simulink library "DC_GRIDSIM_LIB"  (R2022b)
settings: Solver=VariableStepAuto  StartTime=0.0  StopTime=10.0  RelTol=1e-3
undefined symbols (not defined in the file): Allday_timevector, DiscIntNeverNeededParam, High, Household1_Autumnallday, Household1_Springallday, Household1_Summerallday, Household1_Winterallday, Household9_Autumnallday, Household9_Springallday, Household9_Summerallday, Household9_Winterallday, Low, MV, Shift
libraries: fl_lib x66, nesl_utility x33, simulink x8, ee_lib x4
(part 2 of 2)

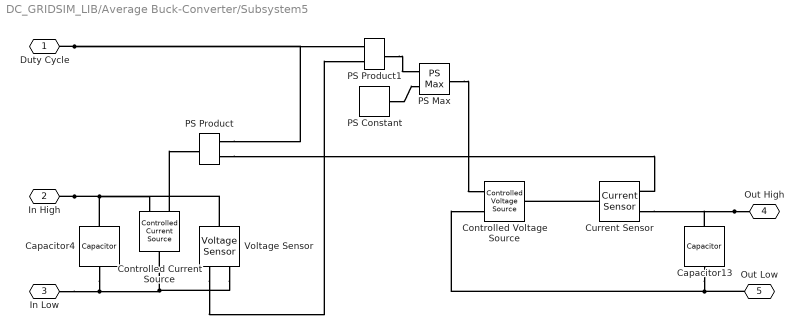
== system DC_GRIDSIM_LIB/Average Buck-Converter/Subsystem5 ==
  Capacitor13 : fl_lib/Electrical/Electrical Elements/Capacitor  c=C uF  r=1e-6 Ohm  g=0 1/Ohm  i_specify=off  i_priority=None  i=1 A  i_nominal_specify=off  i_nominal_unit=A  i_nominal_value=1  v_specify=off  v_priority=None  v=48 V  v_nominal_specify=off  v_nominal_unit=V  v_nominal_value=1  vc_specify=on  vc_priority=None  vc=LV V  vc_nominal_specify=off  vc_nominal_unit=V  vc_nominal_value=1
  Capacitor4 : fl_lib/Electrical/Electrical Elements/Capacitor  c=C uF  r=1e-6 Ohm  g=0 1/Ohm  i_specify=off  i_priority=None  i=1 A  i_nominal_specify=off  i_nominal_unit=A  i_nominal_value=1  v_specify=off  v_priority=High  v=LV V  v_nominal_specify=off  v_nominal_unit=V  v_nominal_value=1  vc_specify=on  vc_priority=None  vc=MV V  vc_nominal_specify=off  vc_nominal_unit=V  vc_nominal_value=1
  Controlled Current Source : fl_lib/Electrical/Electrical Sources/Controlled Current Source
  Controlled Voltage Source : fl_lib/Electrical/Electrical Sources/Controlled Voltage Source
  Current Sensor : fl_lib/Electrical/Electrical Sensors/Current Sensor
  PS Constant : fl_lib/Physical Signals/Sources/PS Constant  constant=1e-3 V
  PS Max : fl_lib/Physical Signals/Nonlinear Operators/PS Max
      settings: InternalSimscapePortConfiguration="{\"Bottom\":[],\"Left\":[{\"id\":\"I1\",\"label\":\"\",\"type\":\"input\"},{\"id\":\"I2\",\"label\":\"\",\"type\":\"input\"}],\"Right\":[{\"id\":\"O\",\"label\":\"\",\"type\":\"output\"}],\"Top\":[]}"
  PS Product : fl_lib/Physical Signals/Functions/PS Product
  PS Product1 : fl_lib/Physical Signals/Functions/PS Product
  Voltage Sensor : fl_lib/Electrical/Electrical Sensors/Voltage Sensor
  Duty Cycle : PMIOPort  Side=Left
  In High : PMIOPort  Port=2  Side=Left
  In Low : PMIOPort  Port=3  Side=Left
  Out High : PMIOPort  Port=4  Side=Right
  Out Low : PMIOPort  Port=5  Side=Right
  connections:
  In High/RConn1 -- Capacitor4/LConn1 -- Voltage Sensor/LConn1 -- Controlled Current Source/RConn2
  In Low/RConn1 -- Capacitor4/RConn1 -- Voltage Sensor/RConn2 -- Controlled Current Source/LConn1
  Duty Cycle/RConn1 -- PS Product/LConn2 -- PS Product1/LConn1
  Out Low/RConn1 -- Capacitor13/RConn1 -- Controlled Voltage Source/RConn2
  Out High/RConn1 -- Current Sensor/RConn2 -- Capacitor13/LConn1
  Current Sensor/LConn1 -- Controlled Voltage Source/LConn1
  PS Constant/RConn1 -- PS Max/LConn2
  Controlled Current Source/RConn1 -- PS Product/RConn1
  Voltage Sensor/RConn1 -- PS Product1/LConn2
  PS Product/LConn1 -- Current Sensor/RConn1
  PS Product1/RConn1 -- PS Max/LConn1
  PS Max/RConn1 -- Controlled Voltage Source/RConn1

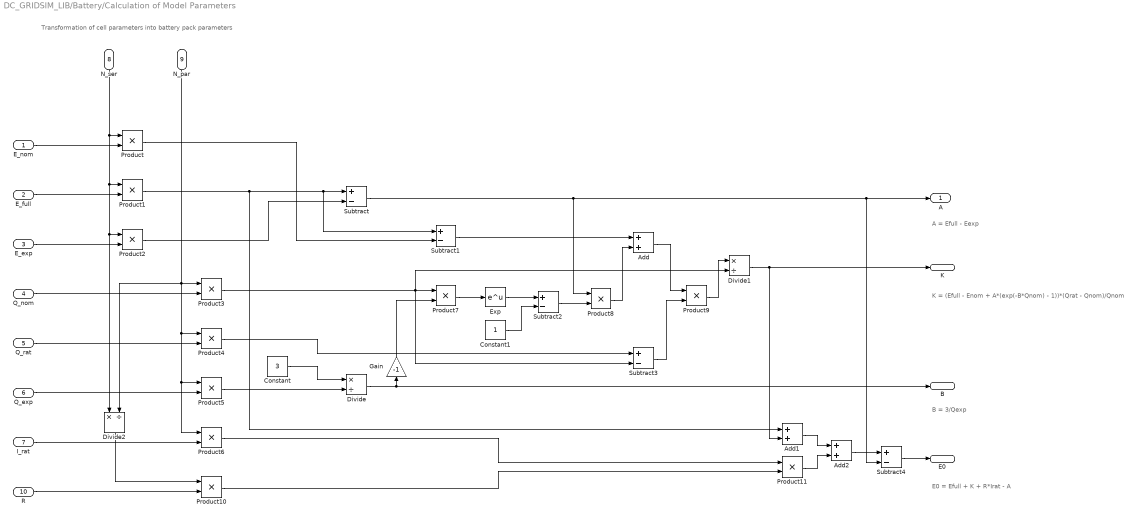
== system DC_GRIDSIM_LIB/Battery/Calculation of Model Parameters ==
  note: A = Efull - Eexp
  note: K = (Efull - Enom + A*(exp(-B*Qnom) - 1))*(Qrat - Qnom)/Qnom
  note: B = 3/Qexp
  note: E0 = Efull + K + R*Irat - A
  note: Transformation of cell parameters into battery pack parameters
  E_nom : Inport
  E_full : Inport  Port=2
  E_exp : Inport  Port=3
  Q_nom : Inport  Port=4
  Q_rat : Inport  Port=5
  Q_exp : Inport  Port=6
  I_rat : Inport  Port=7
  N_ser : Inport  Port=8
  N_par : Inport  Port=9
  R : Inport  Port=10
  Add : Sum
  Add1 : Sum
  Add2 : Sum
  Constant : Constant  Value=3
  Constant1 : Constant
  Divide : Product  Inputs=*/
  Divide1 : Product  Inputs=*/
  Divide2 : Product  Inputs=*/
  Exp : Math
  Gain : Gain  Gain=-1
  Product{,1..11} (12 alike) : Product
  Subtract{,1..4} (5 alike) : Sum  Inputs=+-
  A : Outport
  B : Outport  Port=2
  K : Outport  Port=3
  E0 : Outport  Port=4
  wires:
  Subtract4/1 -> E0/1
  Add2/1 -> Subtract4/1
  Product11/1 -> Add2/2
  Add1/1 -> Add2/1
  Product10/1 -> Product11/2
  Product6/1 -> Product11/1
  Divide2/1 -> Product10/1
  R/1 -> Product10/2
  Divide1/1 -> K/1, Add1/2
  Product9/1 -> Divide1/1
  Subtract3/1 -> Product9/2
  Add/1 -> Product9/1
  Product4/1 -> Subtract3/1
  Product8/1 -> Add/2
  Subtract2/1 -> Product8/2
  Constant1/1 -> Subtract2/2
  Exp/1 -> Subtract2/1
  Subtract1/1 -> Add/1
  Product7/1 -> Exp/1
  Product3/1 -> Product7/1, Divide1/2, Subtract3/2
  Gain/1 -> Product7/2
  Product/1 -> Subtract1/2
  Divide/1 -> Gain/1, B/1
  Product5/1 -> Divide/2
  Constant/1 -> Divide/1
  Subtract/1 -> Product8/1, Subtract4/2, A/1
  Product2/1 -> Subtract/2
  Product1/1 -> Add1/1, Subtract1/1, Subtract/1
  I_rat/1 -> Product6/2
  N_par/1 -> Product6/1, Product5/1, Product4/1, Product3/1, Divide2/2
  Q_exp/1 -> Product5/2
  Q_rat/1 -> Product4/2
  Q_nom/1 -> Product3/2
  E_exp/1 -> Product2/2
  E_full/1 -> Product1/2
  N_ser/1 -> Product/1, Product1/1, Divide2/1, Product2/1
  E_nom/1 -> Product/2

== system DC_GRIDSIM_LIB/WindTurbine/Subsystem1 ==
  In1 : Inport
  Square1 : Math  Operator=pow
  power of 3 : Constant  Value=3
  Out1 : Outport
  wires:
  power of 3/1 -> Square1/2
  Square1/1 -> Out1/1
  In1/1 -> Square1/1

== matlab function DC_GRIDSIM_LIB/BESS/MATLAB Function ==
  data: SOC_init input; SOC output; idt input; Qbat input
function SOC = fcn(SOC_init,idt,Qbat)

SOC = (SOC_init*Qbat+idt)/Qbat;

== matlab function DC_GRIDSIM_LIB/Battery/MATLAB Function1 ==
  data: SOC_init input; A input; B input; K input; E0 input; idt input; Qbat input; E output; SOC output
function [E,SOC] = fcn(SOC_init,A,B,K,E0,idt,Qbat)

it = (1-SOC_init)*Qbat + idt;
E = E0 - K*Qbat/(Qbat-it)+A*exp(-B*it);
SOC = (SOC_init*Qbat-idt)/Qbat;

== matlab function DC_GRIDSIM_LIB/BESS/MATLAB Function1 ==
  data: Pref input; Pbat output; SOC input; SOC_min input; SOC_max input; P_max input
function Pbat = fcn(Pref, SOC, SOC_min, SOC_max, P_max)

if (Pref < 0) && (SOC <= SOC_min)
    Pbat = 0;
elseif (Pref > 0) && (SOC >= SOC_max)
    Pbat = 0;
elseif (Pref > P_max)
    Pbat = P_max;
elseif (Pref < -P_max)
    Pbat = - P_max;
else
    Pbat = Pref;
end

== matlab function DC_GRIDSIM_LIB/Battery/MATLAB Function ==
  data: D_SOC input; Qch output; Qch input; Qdis input; Qrat input; Qdis output
function [Qch,Qdis] = fcn(D_SOC,Qch,Qdis,Qrat)

if D_SOC >= 0
    D_Qch = D_SOC*Qrat;
    Qch = Qch + D_Qch;
else
    D_Qdis = (-1)*D_SOC*Qrat;
    Qdis = Qdis + D_Qdis;
end

== matlab function DC_GRIDSIM_LIB/HouseholdWithFlexibility/MATLAB Function ==
  data: button1 input; button2 input; button3 input; button4 input; data1 input; data2 input; y output; data3 input; data4 input
function y = fcn(button1, button2, button3, button4, data1,data2,data3, data4)
    if button1
        y = data1;
    elseif button2
        y =data2;
    elseif button3
        y = data3;
    elseif button4
        y = data4;
    else 
        y = data1;
    end
end

== matlab function DC_GRIDSIM_LIB/HouseholdWithFlexibility/PeakShaving ==
  data: Power input; PeakShaving input; PeakLimit input; Pload output
function Pload = fcn(Power,PeakShaving,PeakLimit)

% As one option of demand side management, peak shaving can be applied
if (abs(Power) > PeakLimit) && (PeakShaving == 1)
    Pload = PeakLimit;
else
    Pload = Power;
end

== matlab function DC_GRIDSIM_LIB/HouseholdWithFlexibility/MATLAB Function1 ==
  data: Load input; flxLoad output; baseLoad output; Base input; flxQuota input
function [flxLoad, baseLoad] = fcn(Load, Base, flxQuota)

if (Load > Base)
    flxLoad = (Load-Base)*flxQuota;
    baseLoad = Load - flxLoad;
else
    flxLoad = 0;
    baseLoad = Load;
end

== matlab function DC_GRIDSIM_LIB/Household/MATLAB Function ==
  data: button1 input; button2 input; button3 input; button4 input; data1 input; data2 input; y output; data3 input; data4 input
function y = fcn(button1, button2, button3, button4, data1,data2,data3, data4)
    if button1
        y = data1;
    elseif button2
        y =data2;
    elseif button3
        y = data3;
    elseif button4
        y = data4;
    else 
        y = data1;
    end
end
